simulink model "enabled"  (R2014a)
settings: Solver=ode3  StartTime=0.0  StopTime=Inf  RelTol=1e-3
undefined symbols (not defined in the file): DiscIntNeverNeededParam
libraries: simulink x2
settings Model: Creator=eruffaldi  LastModifiedBy=eruffaldi

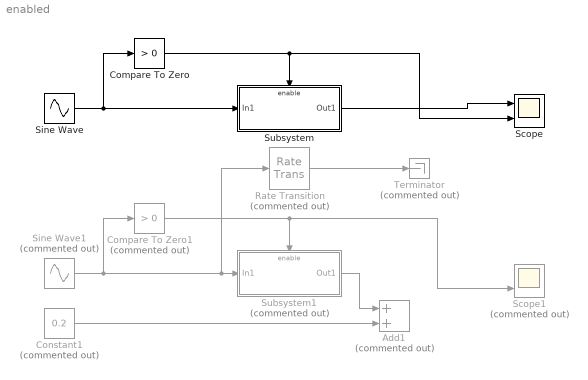
== system enabled ==
  Add1 : Sum  Commented=on
  Compare To Zero : simulink/Logic and Bit Operations/Compare To Zero  relop=>  OutDataTypeStr=boolean
  Compare To Zero1 : simulink/Logic and Bit Operations/Compare To Zero  Commented=on  relop=>  OutDataTypeStr=boolean
  Constant1 : Constant  Commented=on  Value=0.2
  Rate Transition : RateTransition  Commented=on
  Scope : Scope  NumInputPorts=2
      settings: TimeRange=600  YMin=0~0  YMax=2~1
  Scope1 : Scope  Commented=on  NumInputPorts=2
      settings: YMin=-5~-5  YMax=5~5
  Sine Wave : Sin  SampleTime=0.1
  Sine Wave1 : Sin  Commented=on  SampleTime=0.2
  Subsystem : Subsystem
  Subsystem1 : Subsystem  Commented=on
  Terminator : Terminator  Commented=on
  wires:
  Sine Wave/1 -> Subsystem/1(In1), Compare To Zero/1
  Compare To Zero/1 -> Scope/2, Subsystem/Enable
  Subsystem/1(Out1) -> Scope/1
  Sine Wave1/1 -> Rate Transition/1, Subsystem1/1(In1), Compare To Zero1/1
  Compare To Zero1/1 -> Scope1/2, Subsystem1/Enable
  Constant1/1 -> Add1/2
  Subsystem1/1(Out1) -> Add1/1
  Rate Transition/1 -> Terminator/1

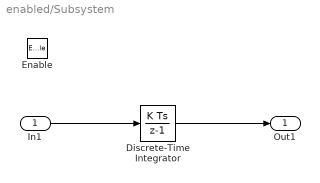
== system enabled/Subsystem ==
  In1 : Inport
  Enable : EnablePort  StatesWhenEnabling=reset
  Discrete-Time Integrator : DiscreteIntegrator  SampleTime=-1  ICPrevOutput=DiscIntNeverNeededParam  ICPrevScaledInput=DiscIntNeverNeededParam
  Out1 : Outport
  wires:
  In1/1 -> Discrete-Time Integrator/1
  Discrete-Time Integrator/1 -> Out1/1

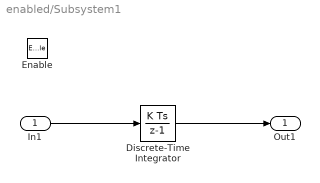
== system enabled/Subsystem1 ==
  In1 : Inport
  Enable : EnablePort
  Discrete-Time Integrator : DiscreteIntegrator  SampleTime=-1  ICPrevOutput=DiscIntNeverNeededParam  ICPrevScaledInput=DiscIntNeverNeededParam
  Out1 : Outport
  wires:
  In1/1 -> Discrete-Time Integrator/1
  Discrete-Time Integrator/1 -> Out1/1
